simulink model "linear_reg_2"  (Simulink 7.4)
settings: Solver=ode45  StartTime=0.0  StopTime=100e-6  MaxStep=1e-6  RelTol=1e-3
undefined symbols (not defined in the file or in its folder): opamp, sigbuilder_block, simpower_extensions_1
libraries: powerlib x17, simulink x3
settings Model: Creator=Owner  LastModifiedBy=Dick
settings OptimizationCC: InitFltsAndDblsToZero=on

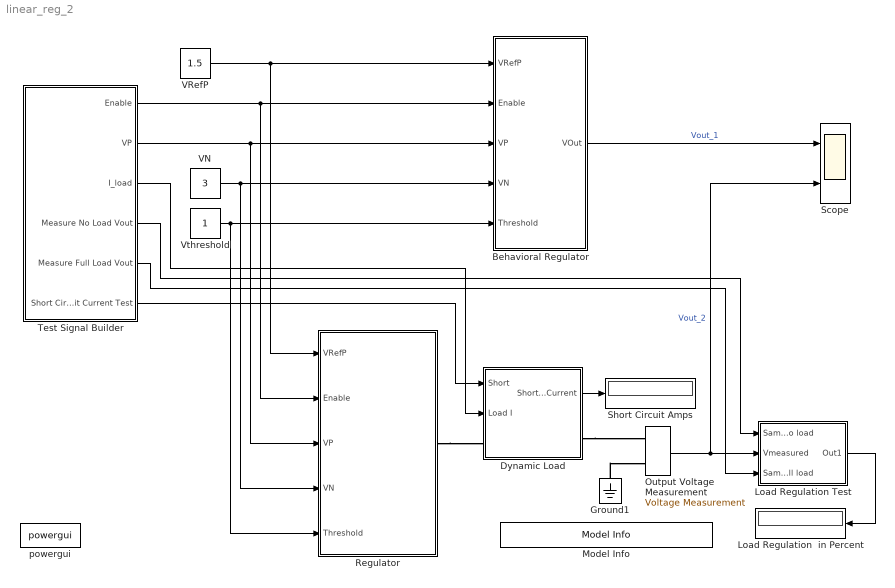
== system linear_reg_2 ==
  Behavioral Regulator : Subsystem
  Dynamic Load : Subsystem
  Ground1 : powerlib/Elements/Ground  DialogController=POWERSYS.PowerSysDialog  PhysicalDomain=powersysdomain  SubClassName=unknown  LeftPortType=p1  RightPortType=p1  LConnTagsString=a
  Load Regulation  in Percent : Display
  Load Regulation Test : Subsystem
  Model Info : simulink/Model-Wide Utilities/Model Info  SystemSampleTime=-1  InitialBlockCM=None  BlockCM=None  Frame=on  DisplayStringWithTags=Copywrite 2005-2010 The MathWorks, Inc.  HorizontalTextAlignment=Center  LeftAlignmentValue=0.5  SourceBlockDiagram=linear_reg_2  TagMaxNumber=20
  Output Voltage  Measurement : powerlib/Measurements/Voltage Measurement  Tag=PoWeRsYsTeMmEaSuReMeNt  DialogController=POWERSYS.PowerSysDialog  SystemSampleTime=-1  PhasorSimulation=off  OutputType=Magnitude  PSBequivalent=0
  Regulator : Subsystem
  Scope : Scope  NumInputPorts=2
      settings: TimeRange=0.00012  YMin=-0.5~-0.5  YMax=3~3
  Short Circuit Amps : Display
  Test Signal Builder : Subsystem  Tag=STV Subsys  LoadFcn=sigbuilder_block('load',[69.75 144 537.75 378.75 ]);  StartFcn=sigbuilder_block('start');  StopFcn=sigbuilder_block('stop');  ClipboardFcn=sigbuilder_block('clipboard');  mask(Sigbuilder block){}
      mask help: Sigbuilder GUI
      mask init:
      | if ~strcmp(get_param(bdroot(gcbh),'SimulationStatus'),'stopped') tuvar = sigbuilder_block('maskInit'); end
      settings: CopyFcn=sigbuilder_block('copy');  DeleteFcn=sigbuilder_block('delete');  ModelCloseFcn=sigbuilder_block('modelClose');  PreSaveFcn=sigbuilder_block('preSave');  NameChangeFcn=sigbuilder_block('namechange');  OpenFcn=sigbuilder_block('open',[437.6 199.2 550.4 400 ]);  CloseFcn=sigbuilder_block('close');
      mask Display: plot(0,0,100,100,[10,10,40,40,10],[80,20,20,80,80],[40,10],[50,50], [40,27,10],[65,72,56],[40,25,25,10],[28,28,43,43]);
  VN : Constant  Value=3  OutDataType=sfix(16)  OutScaling=2^0
  VRefP : Constant  Value=1.5  OutDataType=sfix(16)  OutScaling=2^0
  Vthreshold : Constant  OutDataType=sfix(16)  OutScaling=2^0
  powergui : powerlib/powergui  SystemSampleTime=-1  SimulationMode=Continuous  SampleTime=0  frequency=60  SPID=off  DisableSnubberDevices=off  DisableRonSwitches=off  DisableVfSwitches=off  SwTol=0  Interpol=off  frequencyindice=0  echomessages=off  HookPort=off  DisplayEquations=off  FunctionMessages=off  EnableUseOfTLC=off  x0status=blocks  RestoreLinks=warning  Frange=[0:2:500]  Ylog=off  Xlog=on  ShowGrid=off  save=off  variable=ZData  ZoomFFT=on  StartTime=0.0  cycles=1  DisplayStyle=1  fundamental=60  FreqAxis=off  MaxFrequency=1000  frequencyindicesteady=1  RmsSteady=1  display=off  Ts=0  methode=off
  wires:
  Test Signal Builder/2(VP) -> Behavioral Regulator/3(VP), Regulator/3(VP)
  Test Signal Builder/1(Enable) -> Behavioral Regulator/2(Enable), Regulator/2(Enable)
  Vthreshold/1 -> Behavioral Regulator/5(Threshold), Regulator/5(Threshold)
  VRefP/1 -> Behavioral Regulator/1(VRefP), Regulator/1(VRefP)
  VN/1 -> Behavioral Regulator/4(VN), Regulator/4(VN)
  Behavioral Regulator/1(VOut) -> Scope/1  "Vout_1"
  Output Voltage  Measurement/1 -> Scope/2, Load Regulation Test/2(Vmeasured)  "Vout_2"
  Test Signal Builder/3(I_load) -> Dynamic Load/2(Load I)
  Test Signal Builder/5(Measure Full Load Vout) -> Load Regulation Test/3(Sample full load)
  Load Regulation Test/1(Out1) -> Load Regulation  in Percent/1
  Test Signal Builder/6(Short Circuit Current Test) -> Dynamic Load/1(Short)
  Dynamic Load/1(Short Circuit Current) -> Short Circuit Amps/1
  Test Signal Builder/4(Measure No Load Vout) -> Load Regulation Test/1(Sample no load)
  connections:
  Ground1/LConn1 -- Output Voltage  Measurement/LConn2
  Dynamic Load/RConn1 -- Output Voltage  Measurement/LConn1
  Regulator/RConn1 -- Dynamic Load/LConn1

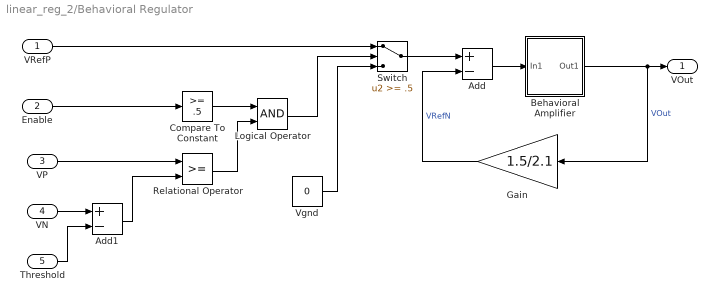
== system linear_reg_2/Behavioral Regulator ==
  VRefP : Inport
  Enable : Inport  Port=2
  VP : Inport  Port=3
  VN : Inport  Port=4
  Threshold : Inport  Port=5
  Add : Sum  Inputs=+-  OutDataType=sfix(16)  OutScaling=2^-10
  Add1 : Sum  Inputs=+-  OutDataType=sfix(16)  OutScaling=2^-10
  Behavioral Amplifier : Subsystem  mask{f2=2e5, f1=1e2, Av=4000, v_min=-3, v_max=3, slew_rate=2e9}
      mask prompts: f2 "break freq 2 in Hz"; f1 "break freq 1 in Hz"; Av "Av (voltage gain)"; v_min "Min Output"; v_max "Max Output"; slew_rate "slew rate (v/s)"
      mask Display: plot([0 1 0 0] , [1 0 -1 1 ]); text(0.15,0.4,'+'); text(0.15,-0.4,'-');
  Compare To Constant : simulink/Logic and Bit Operations/Compare To Constant  SystemSampleTime=-1  relop=>=  const=.5  LogicOutDataTypeMode=boolean  ZeroCross=off
  Gain : Gain  Gain=1.5/2.1  ParameterDataType=sfix(16)  ParameterScaling=2^0  OutDataType=sfix(16)  OutScaling=2^0
  Logical Operator : Logic  AllPortsSameDT=off  OutDataTypeMode=boolean  OutDataTypeStr=boolean
  Relational Operator : RelationalOperator  LogicOutDataTypeMode=boolean  OutDataTypeStr=boolean
  Switch : Switch  Threshold=.5  OutDataType=sfix(16)  OutScaling=2^0
  Vgnd : Constant  Value=0  OutDataType=sfix(16)  OutScaling=2^0
  VOut : Outport
  wires:
  Gain/1 -> Add/2  "VRefN"
  Behavioral Amplifier/1(Out1) -> Gain/1, VOut/1  "VOut"
  Vgnd/1 -> Switch/3
  Logical Operator/1 -> Switch/2
  Compare To Constant/1 -> Logical Operator/1
  Relational Operator/1 -> Logical Operator/2
  Add1/1 -> Relational Operator/2
  Add/1 -> Behavioral Amplifier/1(In1)
  Switch/1 -> Add/1
  VRefP/1 -> Switch/1
  Enable/1 -> Compare To Constant/1
  VP/1 -> Relational Operator/1
  VN/1 -> Add1/1
  Threshold/1 -> Add1/2

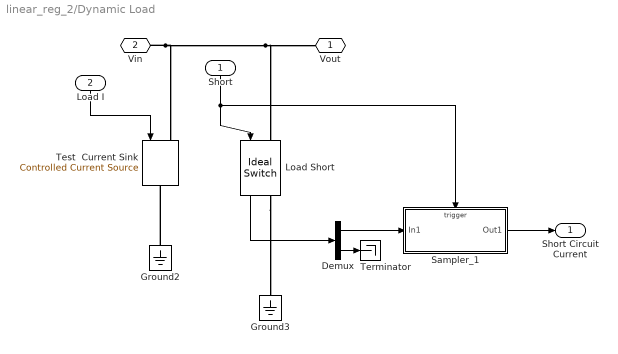
== system linear_reg_2/Dynamic Load ==
  Short : Inport
  Load I : Inport  Port=2
  Demux : Demux  Outputs=2
  Ground2 : powerlib/Elements/Ground  DialogController=POWERSYS.PowerSysDialog  PhysicalDomain=powersysdomain  SubClassName=unknown  LeftPortType=p1  RightPortType=p1  LConnTagsString=a
  Ground3 : powerlib/Elements/Ground  DialogController=POWERSYS.PowerSysDialog  PhysicalDomain=powersysdomain  SubClassName=unknown  LeftPortType=p1  RightPortType=p1  LConnTagsString=a
  Load Short : powerlib/Power Electronics/Ideal Switch  DialogController=POWERSYS.PowerSysDialog  SystemSampleTime=-1  Ron=0.001  Lon=0  IC=0  Rs=1e5  Cs=0  Measurements=on
  Sampler_1 : Subsystem
  Terminator : Terminator
  Test  Current Sink : powerlib/Electrical Sources/Controlled Current Source  DialogController=POWERSYS.PowerSysDialog  SystemSampleTime=-1  Initialize=off  Source_Type=DC  Amplitude=0  Phase=0  Frequency=0  Measurements=None
  Vout : PMIOPort  Port=1  Side=Right
  Vin : PMIOPort  Port=2  Side=Left
  Short Circuit Current : Outport  OutDataType=sfix(16)  OutScaling=2^0
  wires:
  Short/1 -> Load Short/1, Sampler_1/Trigger
  Load I/1 -> Test  Current Sink/1
  Load Short/1 -> Demux/1
  Demux/2 -> Terminator/1
  Demux/1 -> Sampler_1/1(In1)
  Sampler_1/1(Out1) -> Short Circuit Current/1
  connections:
  Ground2/LConn1 -- Test  Current Sink/RConn1
  Load Short/RConn1 -- Ground3/LConn1
  Vin/RConn1 -- Load Short/LConn1 -- Vout/RConn1 -- Test  Current Sink/LConn1

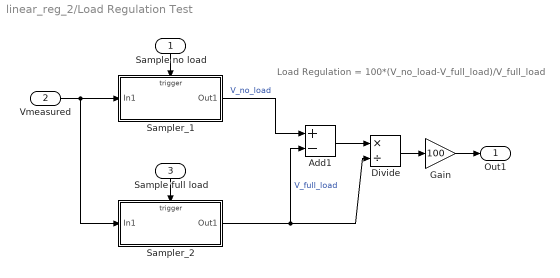
== system linear_reg_2/Load Regulation Test ==
  note: Load Regulation = 100*(V_no_load-V_full_load)/V_full_load
  Sample no load : Inport
  Vmeasured : Inport  Port=2
  Sample full load : Inport  Port=3
  Add1 : Sum  Inputs=+-  OutDataType=sfix(16)  OutScaling=2^-10
  Divide : Product  Inputs=*/  OutDataType=sfix(16)  OutScaling=2^-10
  Gain : Gain  Gain=100  ParameterDataType=sfix(16)  ParameterScaling=2^0  OutDataType=sfix(16)  OutScaling=2^0
  Sampler_1 : Subsystem
  Sampler_2 : Subsystem
  Out1 : Outport
  wires:
  Sampler_1/1(Out1) -> Add1/1  "V_no_load"
  Sampler_2/1(Out1) -> Add1/2, Divide/2  "V_full_load"
  Add1/1 -> Divide/1
  Divide/1 -> Gain/1
  Vmeasured/1 -> Sampler_1/1(In1), Sampler_2/1(In1)
  Sample no load/1 -> Sampler_1/Trigger
  Sample full load/1 -> Sampler_2/Trigger
  Gain/1 -> Out1/1

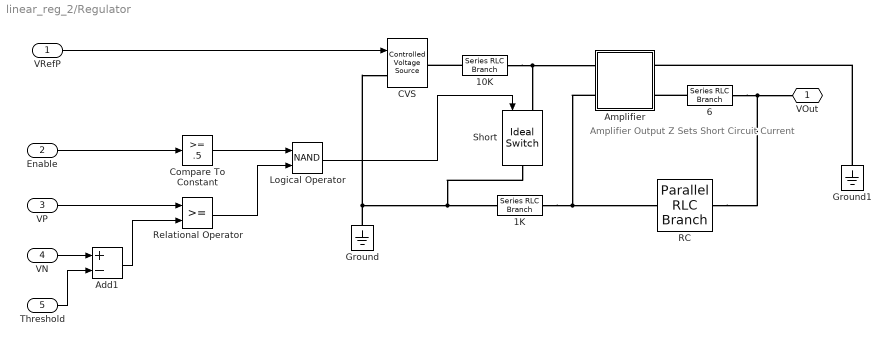
== system linear_reg_2/Regulator ==
  note: Amplifier Output Z
      | Sets Short Circuit Current
  VRefP : Inport
  Enable : Inport  Port=2
  VP : Inport  Port=3
  VN : Inport  Port=4
  Threshold : Inport  Port=5
  10K : powerlib/Elements/Series RLC Branch  DialogController=POWERSYS.PowerSysDialog  PhysicalDomain=powersysdomain  SubClassName=unknown  LeftPortType=p1  RightPortType=p1  LConnTagsString=__new0  RConnTagsString=__new0  BranchType=R  Resistance=10000  Inductance=1.0  SetiL0=off  InitialCurrent=0  Capacitance=1.0  Setx0=off  InitialVoltage=0  Measurements=None
  1K : powerlib/Elements/Series RLC Branch  DialogController=POWERSYS.PowerSysDialog  PhysicalDomain=powersysdomain  SubClassName=unknown  LeftPortType=p1  RightPortType=p1  LConnTagsString=__new0  RConnTagsString=__new0  BranchType=R  Resistance=1000  Inductance=1.0  SetiL0=off  InitialCurrent=0  Capacitance=1.0  Setx0=off  InitialVoltage=0  Measurements=None
  6 : powerlib/Elements/Series RLC Branch  DialogController=POWERSYS.PowerSysDialog  PhysicalDomain=powersysdomain  SubClassName=unknown  LeftPortType=p1  RightPortType=p1  LConnTagsString=__new0  RConnTagsString=__new0  BranchType=R  Resistance=6  Inductance=1.0  SetiL0=off  InitialCurrent=0  Capacitance=1.0  Setx0=off  InitialVoltage=0  Measurements=None
  Add1 : Sum  Inputs=+-  OutDataType=sfix(16)  OutScaling=2^-10
  Amplifier : Subsystem  AncestorBlock=simpower_extensions_1/opamp  mask{f2=2e5, f1=1e2, Av=4000, v_min=-3, v_max=3, slew_rate=2e9}
      mask prompts: f2 "break freq 2 in Hz"; f1 "break freq 1 in Hz"; Av "Av (voltage gain)"; v_min "Min Output"; v_max "Max Output"; slew_rate "slew rate (v/s)"
      mask Display: plot([0 1 0 0] , [1 0 -1 1 ]); text(0.15,0.4,'+'); text(0.15,-0.4,'-');
  CVS : powerlib/Electrical Sources/Controlled Voltage Source  Description=source block  DialogController=POWERSYS.PowerSysDialog  SystemSampleTime=-1  Initialize=off  Source_Type=AC  Amplitude=0  Phase=0  Frequency=0  Measurements=None
      settings: AttributesFormatString=\n
  Compare To Constant : simulink/Logic and Bit Operations/Compare To Constant  SystemSampleTime=-1  relop=>=  const=.5  LogicOutDataTypeMode=boolean  ZeroCross=off
  Ground : powerlib/Elements/Ground  DialogController=POWERSYS.PowerSysDialog  PhysicalDomain=powersysdomain  SubClassName=unknown  LeftPortType=p1  RightPortType=p1  LConnTagsString=a
  Ground1 : powerlib/Elements/Ground  DialogController=POWERSYS.PowerSysDialog  PhysicalDomain=powersysdomain  SubClassName=unknown  LeftPortType=p1  RightPortType=p1  LConnTagsString=a
  Logical Operator : Logic  Operator=NAND  AllPortsSameDT=off  OutDataTypeMode=boolean  OutDataTypeStr=boolean
  RC : powerlib/Elements/Parallel RLC Branch  DialogController=POWERSYS.PowerSysDialog  PhysicalDomain=powersysdomain  SubClassName=unknown  LeftPortType=p1  RightPortType=p1  LConnTagsString=a  RConnTagsString=__new0  BranchType=RC  Resistance=1000*(2.1/1.5 - 1)  Inductance=1.0  SetiL0=off  InitialCurrent=0  Capacitance=2e-9  Setx0=off  InitialVoltage=0  Measurements=None
  Relational Operator : RelationalOperator  LogicOutDataTypeMode=boolean  OutDataTypeStr=boolean
  Short : powerlib/Power Electronics/Ideal Switch  DialogController=POWERSYS.PowerSysDialog  SystemSampleTime=-1  Ron=0.001  Lon=0  IC=0  Rs=1e5  Cs=0  Measurements=off
  VOut : PMIOPort  Port=1  Side=Right
  wires:
  VRefP/1 -> CVS/1
  Logical Operator/1 -> Short/1
  Compare To Constant/1 -> Logical Operator/1
  Relational Operator/1 -> Logical Operator/2
  Add1/1 -> Relational Operator/2
  Enable/1 -> Compare To Constant/1
  VP/1 -> Relational Operator/1
  VN/1 -> Add1/1
  Threshold/1 -> Add1/2
  connections:
  Ground/LConn1 -- CVS/LConn1 -- 1K/LConn1 -- Short/RConn1
  1K/RConn1 -- Amplifier/LConn2 -- RC/LConn1
  6/LConn1 -- Amplifier/RConn2
  6/RConn1 -- RC/RConn1 -- VOut/RConn1
  Ground1/LConn1 -- Amplifier/RConn1
  10K/LConn1 -- CVS/RConn1
  10K/RConn1 -- Amplifier/LConn1 -- Short/LConn1

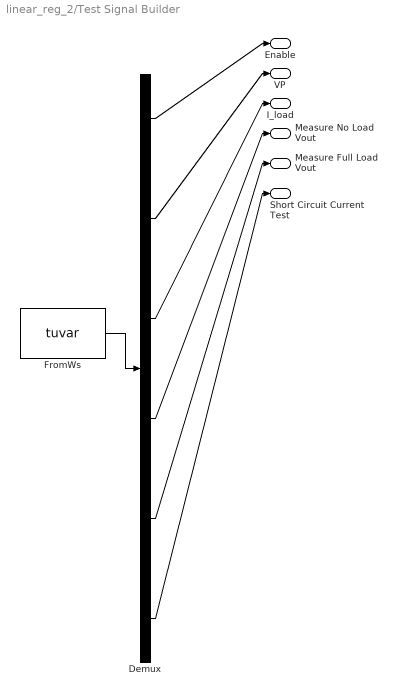
== system linear_reg_2/Test Signal Builder ==
  Demux : Demux  Tag=STV Demux  Outputs=6
  FromWs : FromWorkspace  Tag=STV FromWs  VariableName=tuvar  SampleTime=0  SigBuilderData=DataTag0  VnvData=DataTag1
      SigBuilderData=|
      | common.afterFinalStr = 'Extrapolate'
      | common.sampleTime = 0
      | dataSet.timeRange = [0 0.0001]
      | dataSet.name = 'Group 1'
      | sbobj.Groups.Name = 'Group 1'
      | sbobj.Groups.Signals(1).Name = 'Enable'
      | sbobj.Groups.Signals(1).XData = [0 2.5e-06 2.5e-06 9e-05 9e-05 0.0001]
      | sbobj.Groups.Signals(1).YData = [0 0 1 1 0 0]
      | sbobj.Groups.Signals(2).Name = 'VP'
      | sbobj.Groups.Signals(2).XData = [0 4.5e-06 5.1e-06 1.12e-05 4.06e-05 0.0001]
      | sbobj.Groups.Signals(2).YData = [0 -0.05 0.2 3.05 3 3]
      | sbobj.Groups.Signals(3).Name = 'I_load'
      | sbobj.Groups.Signals(3).XData = [0 3e-05 3e-05 4.98e-05 4.98e-05 0.0001]
      | sbobj.Groups.Signals(3).YData = [0 0 0.1 0.1 0 0]
      | sbobj.Groups.Signals(4).Name = 'Measure No Load Vout'
      | sbobj.Groups.Signals(4).XData = [0 2.9e-05 2.9e-05 2.96e-05 2.96e-05 0.0001]
      | sbobj.Groups.Signals(4).YData = [0 0 1 1 0 0]
      | sbobj.Groups.Signals(5).Name = 'Measure Full Load Vout'
      | sbobj.Groups.Signals(5).XData = [0 4.77e-05 4.77e-05 4.82e-05 4.82e-05 0.0001]
      | sbobj.Groups.Signals(5).YData = [0 0 1 1 0 0]
      | sbobj.Groups.Signals(6).Name = 'Short Circuit Current Test'
      | sbobj.Groups.Signals(6).XData = [0 6.99e-05 6.99e-05 7.24e-05 7.24e-05 0.0001]
      | sbobj.Groups.Signals(6).YData = [0 0 1 1 0 0]
  Enable : Outport  Tag=STV Outport  OutDataType=sfix(16)  OutScaling=2^0
  VP : Outport  Tag=STV Outport  Port=2
  I_load : Outport  Tag=STV Outport  Port=3
  Measure No Load Vout : Outport  Tag=STV Outport  Port=4
  Measure Full Load Vout : Outport  Tag=STV Outport  Port=5
  Short Circuit Current Test : Outport  Tag=STV Outport  Port=6
  wires:
  FromWs/1 -> Demux/1
  Demux/1 -> Enable/1
  Demux/2 -> VP/1
  Demux/3 -> I_load/1
  Demux/4 -> Measure No Load Vout/1
  Demux/5 -> Measure Full Load Vout/1
  Demux/6 -> Short Circuit Current Test/1

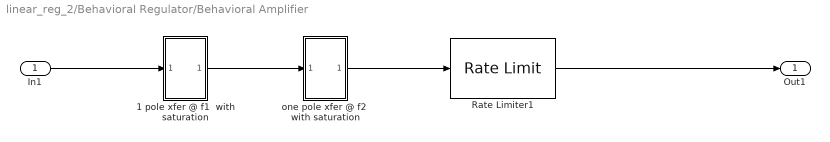
== system linear_reg_2/Behavioral Regulator/Behavioral Amplifier ==
  In1 : Inport  OutDataType=sfix(16)  OutScaling=2^0
  1 pole xfer @ f1  with saturation : Subsystem
  Rate Limiter1 : RateLimiter  RisingSlewLimit=slew_rate  FallingSlewLimit=-slew_rate  LinearizeAsGain=off
  one pole xfer @ f2  with saturation : Subsystem
  Out1 : Outport  OutDataType=sfix(16)  OutScaling=2^0
  wires:
  Rate Limiter1/1 -> Out1/1
  one pole xfer @ f2  with saturation/1(Out1) -> Rate Limiter1/1
  In1/1 -> 1 pole xfer @ f1  with saturation/1(In1)
  1 pole xfer @ f1  with saturation/1(Out1) -> one pole xfer @ f2  with saturation/1(In1)

== system linear_reg_2/Dynamic Load/Sampler_1 ==
  In1 : Inport  OutDataType=sfix(16)  OutScaling=2^0
  Trigger : TriggerPort  TriggerType=falling
  Out1 : Outport  OutDataType=sfix(16)  OutScaling=2^0
  wires:
  In1/1 -> Out1/1

== system linear_reg_2/Load Regulation Test/Sampler_1 ==
  In1 : Inport  OutDataType=sfix(16)  OutScaling=2^0
  Trigger : TriggerPort
  Out1 : Outport  OutDataType=sfix(16)  OutScaling=2^0
  wires:
  In1/1 -> Out1/1

== system linear_reg_2/Load Regulation Test/Sampler_2 ==
  In1 : Inport  OutDataType=sfix(16)  OutScaling=2^0
  Trigger : TriggerPort
  Out1 : Outport  OutDataType=sfix(16)  OutScaling=2^0  InitialOutput=eps
  wires:
  In1/1 -> Out1/1

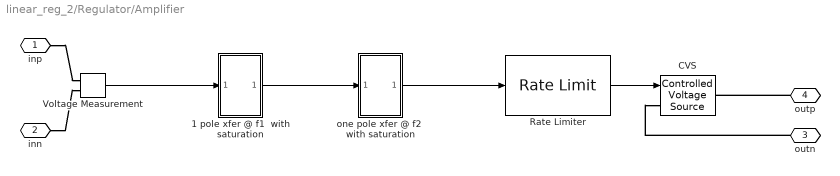
== system linear_reg_2/Regulator/Amplifier ==
  1 pole xfer @ f1  with saturation : Subsystem
  CVS : powerlib/Electrical Sources/Controlled Voltage Source  Description=source block  DialogController=POWERSYS.PowerSysDialog  SystemSampleTime=-1  Initialize=off  Source_Type=AC  Amplitude=0  Phase=0  Frequency=0  Measurements=None
      settings: AttributesFormatString=\n
  Rate Limiter : RateLimiter  RisingSlewLimit=slew_rate  FallingSlewLimit=-slew_rate  LinearizeAsGain=off
  Voltage Measurement : powerlib/Measurements/Voltage Measurement  Tag=PoWeRsYsTeMmEaSuReMeNt  DialogController=POWERSYS.PowerSysDialog  SystemSampleTime=-1  PhasorSimulation=off  OutputType=Magnitude  PSBequivalent=0
  one pole xfer @ f2  with saturation : Subsystem
  inp : PMIOPort  Port=1  Side=Left
  inn : PMIOPort  Port=2  Side=Left
  outn : PMIOPort  Port=3  Side=Right
  outp : PMIOPort  Port=4  Side=Right
  wires:
  Rate Limiter/1 -> CVS/1
  one pole xfer @ f2  with saturation/1(Out1) -> Rate Limiter/1
  Voltage Measurement/1 -> 1 pole xfer @ f1  with saturation/1(In1)
  1 pole xfer @ f1  with saturation/1(Out1) -> one pole xfer @ f2  with saturation/1(In1)
  connections:
  outn/RConn1 -- CVS/LConn1
  inn/RConn1 -- Voltage Measurement/LConn2
  outp/RConn1 -- CVS/RConn1
  inp/RConn1 -- Voltage Measurement/LConn1

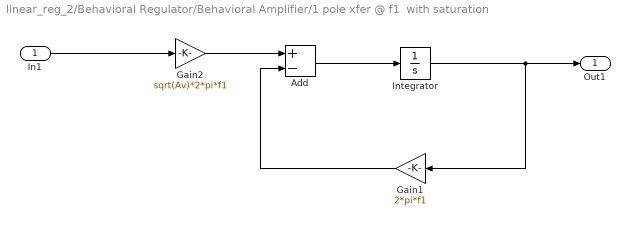
== system linear_reg_2/Behavioral Regulator/Behavioral Amplifier/1 pole xfer @ f1  with saturation ==
  In1 : Inport
  Add : Sum  Inputs=+-  OutDataType=sfix(16)  OutScaling=2^-10
  Gain1 : Gain  Gain=2*pi*f1  ParameterDataType=sfix(16)  ParameterScaling=2^0  OutDataType=sfix(16)  OutScaling=2^0
  Gain2 : Gain  Gain=sqrt(Av)*2*pi*f1  ParameterDataType=sfix(16)  ParameterScaling=2^0  OutDataType=sfix(16)  OutScaling=2^0
  Integrator : Integrator  LimitOutput=on  UpperSaturationLimit=v_max  LowerSaturationLimit=v_min
  Out1 : Outport
  wires:
  Add/1 -> Integrator/1
  Gain1/1 -> Add/2
  Integrator/1 -> Out1/1, Gain1/1
  In1/1 -> Gain2/1
  Gain2/1 -> Add/1

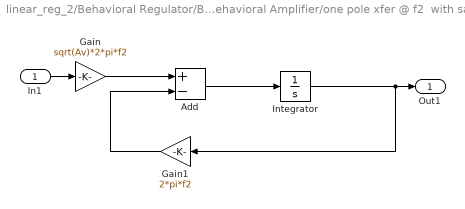
== system linear_reg_2/Behavioral Regulator/Behavioral Amplifier/one pole xfer @ f2  with saturation ==
  In1 : Inport
  Add : Sum  Inputs=+-  OutDataType=sfix(16)  OutScaling=2^-10
  Gain : Gain  Gain=sqrt(Av)*2*pi*f2  ParameterDataType=sfix(16)  ParameterScaling=2^0  OutDataType=sfix(16)  OutScaling=2^0
  Gain1 : Gain  Gain=2*pi*f2  ParameterDataType=sfix(16)  ParameterScaling=2^0  OutDataType=sfix(16)  OutScaling=2^0
  Integrator : Integrator  LimitOutput=on  UpperSaturationLimit=v_max  LowerSaturationLimit=v_min
  Out1 : Outport
  wires:
  In1/1 -> Gain/1
  Integrator/1 -> Out1/1, Gain1/1
  Gain1/1 -> Add/2
  Gain/1 -> Add/1
  Add/1 -> Integrator/1

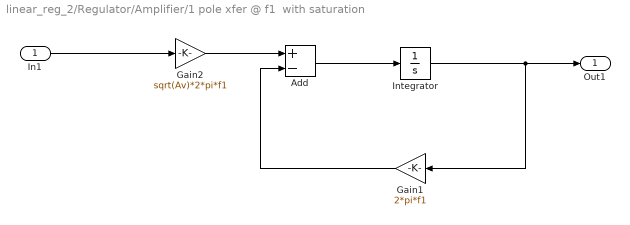
== system linear_reg_2/Regulator/Amplifier/1 pole xfer @ f1  with saturation ==
  In1 : Inport
  Add : Sum  Inputs=+-  OutDataType=sfix(16)  OutScaling=2^-10
  Gain1 : Gain  Gain=2*pi*f1  ParameterDataType=sfix(16)  ParameterScaling=2^0  OutDataType=sfix(16)  OutScaling=2^0
  Gain2 : Gain  Gain=sqrt(Av)*2*pi*f1  ParameterDataType=sfix(16)  ParameterScaling=2^0  OutDataType=sfix(16)  OutScaling=2^0
  Integrator : Integrator  LimitOutput=on  UpperSaturationLimit=v_max  LowerSaturationLimit=v_min
  Out1 : Outport
  wires:
  Add/1 -> Integrator/1
  Gain1/1 -> Add/2
  Integrator/1 -> Out1/1, Gain1/1
  In1/1 -> Gain2/1
  Gain2/1 -> Add/1

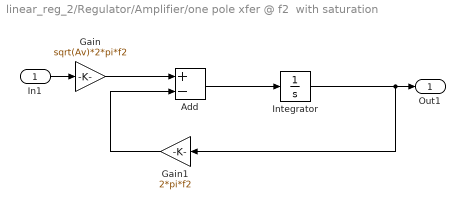
== system linear_reg_2/Regulator/Amplifier/one pole xfer @ f2  with saturation ==
  In1 : Inport
  Add : Sum  Inputs=+-  OutDataType=sfix(16)  OutScaling=2^-10
  Gain : Gain  Gain=sqrt(Av)*2*pi*f2  ParameterDataType=sfix(16)  ParameterScaling=2^0  OutDataType=sfix(16)  OutScaling=2^0
  Gain1 : Gain  Gain=2*pi*f2  ParameterDataType=sfix(16)  ParameterScaling=2^0  OutDataType=sfix(16)  OutScaling=2^0
  Integrator : Integrator  LimitOutput=on  UpperSaturationLimit=v_max  LowerSaturationLimit=v_min
  Out1 : Outport
  wires:
  In1/1 -> Gain/1
  Integrator/1 -> Out1/1, Gain1/1
  Gain1/1 -> Add/2
  Gain/1 -> Add/1
  Add/1 -> Integrator/1
